simulink model "Funcion_transferencia_Simulink"  (R2020b)
settings: Solver=VariableStepAuto  StartTime=0.0  StopTime=100  RelTol=1e-3
undefined symbols (not defined in the file): B, Bm, Jm, K, K1, K2, Kb, kD, Kp, KR, L1, L2, R, wo
settings Model: Creator=Marco  LastModifiedBy=Marco

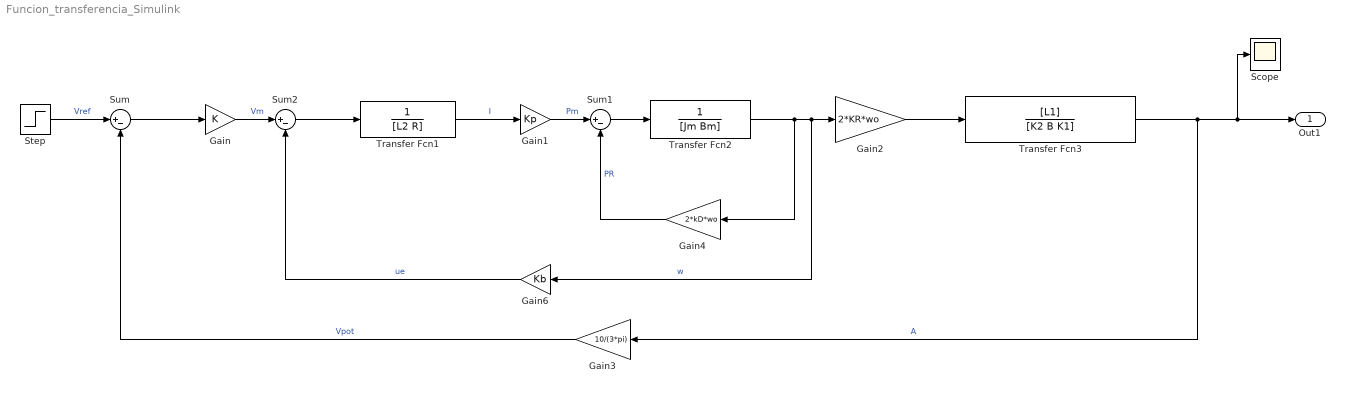
== system Funcion_transferencia_Simulink ==
  Gain : Gain  Gain=K
  Gain1 : Gain  Gain=Kp
  Gain2 : Gain  Gain=2*KR*wo
  Gain3 : Gain  Gain=10/(3*pi)
  Gain4 : Gain  Gain=2*kD*wo
  Gain6 : Gain  Gain=Kb
  Scope : Scope
  Step : Step  SampleTime=0
  Sum : Sum  Inputs=|+-
  Sum1 : Sum  Inputs=|+-
  Sum2 : Sum  Inputs=|+-
  Transfer Fcn1 : TransferFcn  Denominator=[L2 R]
  Transfer Fcn2 : TransferFcn  Denominator=[Jm Bm]
  Transfer Fcn3 : TransferFcn  Numerator=[L1]  Denominator=[K2 B K1]
  Out1 : Outport
  wires:
  Sum1/1 -> Transfer Fcn2/1
  Gain1/1 -> Sum1/1  "Pm"
  Transfer Fcn2/1 -> Gain6/1, Gain2/1, Gain4/1  "w"
  Gain3/1 -> Sum/2  "Vpot"
  Gain2/1 -> Transfer Fcn3/1
  Sum/1 -> Gain/1
  Gain/1 -> Sum2/1  "Vm"
  Gain4/1 -> Sum1/2  "PR"
  Transfer Fcn1/1 -> Gain1/1  "I"
  Gain6/1 -> Sum2/2  "ue"
  Sum2/1 -> Transfer Fcn1/1
  Transfer Fcn3/1 -> Scope/1, Out1/1, Gain3/1  "A"
  Step/1 -> Sum/1  "Vref"
